simulink model "ac_sincos"  (Simulink 9.0)
settings: Solver=FixedStepDiscrete  StartTime=0.0  StopTime=10.0  FixedStep=.00244140625  RelTol=1e-3
libraries: simulink x3, catapult_blocks_lib x1
settings Model: SuppressorTable=22 serialization::archive 11 0 6 0 0 0 11 0  Creator=kharer  LastModifiedBy=kharer
settings DataIOCC: SaveFormat=Dataset
settings OptimizationCC: LifeSpan=auto
settings DebuggingCC: UnderspecifiedInitializationDetection=Simplified  MergeDetectMultiDrivingBlocksExec=error  SFUnexpectedBacktrackingDiag=error  SFNoUnconditionalDefaultTransitionDiag=error  SFExecutionAtInitializationDiag=warning
settings HardwareCC: ProdBitPerPointer=64  ProdBitPerSizeT=64  ProdBitPerPtrDiffT=64  ProdLargestAtomicFloat=Float  ProdIntDivRoundTo=Zero  ProdEndianess=LittleEndian  ProdWordSize=64  ProdHWDeviceType=Intel->x86-64 (Windows64)
settings ModelReferenceCC: PropagateSignalLabelsOutOfModel=on
settings CodeAppCC: StateflowObjectComments=off
settings GRTTargetCC: TargetLangStandard=C99 (ISO)
settings ConfigComp: CovMetricSettings=dwe  CovHtmlReporting=off  CovSaveCumulativeToWorkspaceVar=off  CovSaveSingleToWorkspaceVar=off  CovExternalEMLEnable=on

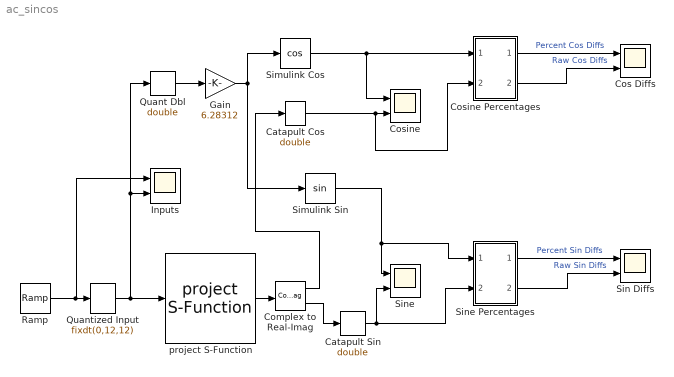
== system ac_sincos ==
  Catapult Cos : DataTypeConversion  OutDataTypeStr=double  RndMeth=Round
  Catapult Sin : DataTypeConversion  OutDataTypeStr=double  RndMeth=Round
  Complex to Real-Imag : ComplexToRealImag
  Cos Diffs : Scope  NumInputPorts=2
  Cosine : Scope  NumInputPorts=2
  Cosine Percentages : Subsystem
  Gain : Gain  Gain=6.28312
  Inputs : Scope  NumInputPorts=2
  Quant Dbl : DataTypeConversion  OutDataTypeStr=double  RndMeth=Round
  Quantized Input : DataTypeConversion  OutDataTypeStr=fixdt(0,12,12)  RndMeth=Round
  Ramp : simulink/Sources/Ramp  slope=0.099  start=0  X0=0
  Simulink Cos : Trigonometry  Operator=cos
  Simulink Sin : Trigonometry
  Sin Diffs : Scope  NumInputPorts=2
  Sine : Scope  NumInputPorts=2
  Sine Percentages : Subsystem
  project S-Function : catapult_blocks_lib/project S-Function  Description=|
      | Description S-Function wrapper around the Catapult C++ function 'project'.
      | Catapult project file: '/wv/fv_engr/kevin/space/matlab/Catapult.ccs'
  wires:
  Quantized Input/1 -> project S-Function/1, Quant Dbl/1, Inputs/2
  project S-Function/1 -> Complex to Real-Imag/1
  Complex to Real-Imag/1 -> Catapult Cos/1
  Complex to Real-Imag/2 -> Catapult Sin/1
  Ramp/1 -> Inputs/1, Quantized Input/1
  Gain/1 -> Simulink Sin/1, Simulink Cos/1
  Sine Percentages/1(Out1) -> Sin Diffs/1  "Percent Sin Diffs"
  Simulink Cos/1 -> Cosine Percentages/1(In1), Cosine/1
  Catapult Cos/1 -> Cosine Percentages/2(In2), Cosine/2
  Simulink Sin/1 -> Sine Percentages/1(In1), Sine/1
  Catapult Sin/1 -> Sine Percentages/2(In2), Sine/2
  Cosine Percentages/1(Out1) -> Cos Diffs/1  "Percent Cos Diffs"
  Cosine Percentages/2(Out2) -> Cos Diffs/2  "Raw Cos Diffs"
  Sine Percentages/2(Out2) -> Sin Diffs/2  "Raw Sin Diffs"
  Quant Dbl/1 -> Gain/1

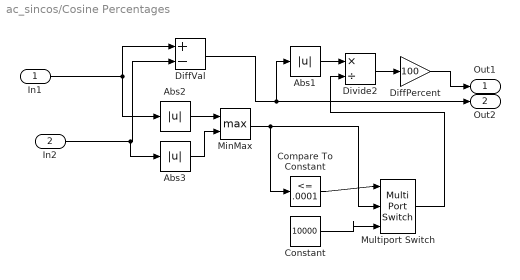
== system ac_sincos/Cosine Percentages ==
  In1 : Inport
  In2 : Inport  Port=2
  Abs1 : Abs
  Abs2 : Abs
  Abs3 : Abs
  Compare To Constant : simulink/Logic and Bit Operations/Compare To Constant  relop=<=  const=.0001  OutDataTypeStr=uint8
  Constant : Constant  Value=10000
  DiffPercent : Gain  Gain=100
  DiffVal : Sum  Inputs=+-
  Divide2 : Product  Inputs=*/
  MinMax : MinMax  Function=max  Inputs=2
  Multiport Switch : MultiPortSwitch  DataPortOrder=Zero-based contiguous  Inputs=2  RndMeth=Round  SaturateOnIntegerOverflow=on  InputSameDT=on
  Out1 : Outport
  Out2 : Outport  Port=2
  wires:
  DiffPercent/1 -> Out1/1
  DiffVal/1 -> Out2/1, Abs1/1
  Divide2/1 -> DiffPercent/1
  Abs2/1 -> MinMax/1
  Abs1/1 -> Divide2/1
  Abs3/1 -> MinMax/2
  Constant/1 -> Multiport Switch/3
  Multiport Switch/1 -> Divide2/2
  MinMax/1 -> Multiport Switch/2, Compare To Constant/1
  Compare To Constant/1 -> Multiport Switch/1
  In2/1 -> DiffVal/2, Abs3/1
  In1/1 -> DiffVal/1, Abs2/1

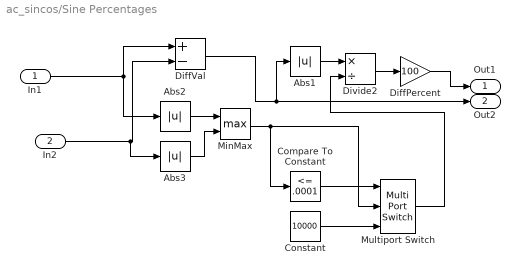
== system ac_sincos/Sine Percentages ==
  In1 : Inport
  In2 : Inport  Port=2
  Abs1 : Abs
  Abs2 : Abs
  Abs3 : Abs
  Compare To Constant : simulink/Logic and Bit Operations/Compare To Constant  relop=<=  const=.0001  OutDataTypeStr=uint8
  Constant : Constant  Value=10000
  DiffPercent : Gain  Gain=100
  DiffVal : Sum  Inputs=+-
  Divide2 : Product  Inputs=*/
  MinMax : MinMax  Function=max  Inputs=2
  Multiport Switch : MultiPortSwitch  DataPortOrder=Zero-based contiguous  Inputs=2  RndMeth=Round  SaturateOnIntegerOverflow=on  InputSameDT=on
  Out1 : Outport
  Out2 : Outport  Port=2
  wires:
  DiffPercent/1 -> Out1/1
  DiffVal/1 -> Out2/1, Abs1/1
  Divide2/1 -> DiffPercent/1
  Abs2/1 -> MinMax/1
  Abs1/1 -> Divide2/1
  Abs3/1 -> MinMax/2
  Constant/1 -> Multiport Switch/3
  Multiport Switch/1 -> Divide2/2
  MinMax/1 -> Multiport Switch/2, Compare To Constant/1
  Compare To Constant/1 -> Multiport Switch/1
  In2/1 -> DiffVal/2, Abs3/1
  In1/1 -> DiffVal/1, Abs2/1
